simulink model "Planar_robot_3DoF_sim"  (R2023a)
settings: Solver=ode3  StartTime=0.0  StopTime=5  FixedStep=0.001  RelTol=1e-3
values from neighbouring files (symbols this model uses):
  amplitude = 20 + 20 * rand(1, num_links)'    [script.m]
  arm_length = [2 2 2]    [script.m]
  freq = 10 + 10 * rand(1, num_links)'    [script.m]
  radius = 0.00002    (= 2e-05)    [script.m]
  rho = 10000000    [script.m]
settings Model: Creator=wu_xw  LastModifiedBy=divij
settings SolverCC: AlgebraicLoopSolver=TrustRegion
settings DataIOCC: SaveFormat=Structure  SaveOutput=off  SignalLogging=off  DSMLogging=off  SaveTime=off  ReturnWorkspaceOutputs=off
settings OptimizationCC: DefaultParameterBehavior=Inlined  UseDivisionForNetSlopeComputation=on  GainParamInheritBuiltInType=on  UseFloatMulNetSlope=on  InlineInvariantSignals=on  ZeroExternalMemoryAtStartup=off  ZeroInternalMemoryAtStartup=off  EfficientFloat2IntCast=on  LifeSpan=1  OptimizeDataStoreBuffers=off  BusAssignmentInplaceUpdate=off
settings DebuggingCC: UnconnectedInputMsg=warning  UnconnectedOutputMsg=warning  UnconnectedLineMsg=warning  SFUnexpectedBacktrackingDiag=warning  SFNoUnconditionalDefaultTransitionDiag=warning  ArithmeticOperatorsInVariantConditions=warning
settings HardwareCC: ProdLongLongMode=on
settings ModelReferenceCC: EnableRefExpFcnMdlSchedulingChecks=on
settings SFSimCC: SimUseLocalCustomCode=off  MATLABDynamicMemAlloc=off  CustomCodeUndefinedFunction=UseInterfaceOnly
settings RTWCC: GenCodeOnly=on  PackageGeneratedCodeAndArtifacts=on  GenerateReport=on  RTWUseLocalCustomCode=off  Toolchain=Catkin  BuildConfiguration=Debug  LaunchReport=on  TargetLang=C++
settings CodeAppCC: ForceParamTrailComments=on  EnableCustomComments=on
settings GRTTargetCC: TargetLangStandard=C++11 (ISO)  CombineSignalStateStructs=on  MatFileLogging=off  CodeInterfacePackaging=C++ class  SupportVariableSizeSignals=on  MultiInstanceErrorCode=Warning

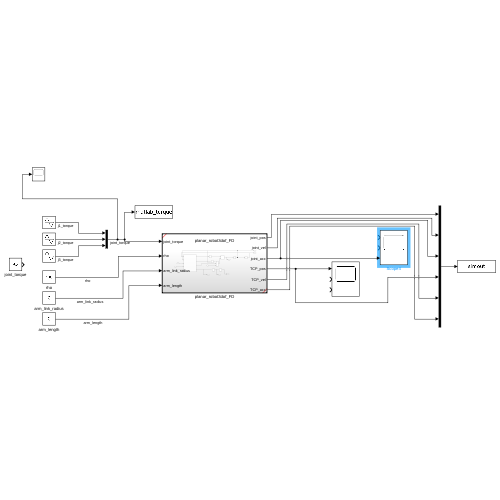
[thumbnail: Simulink's stored preview of the top-level diagram]
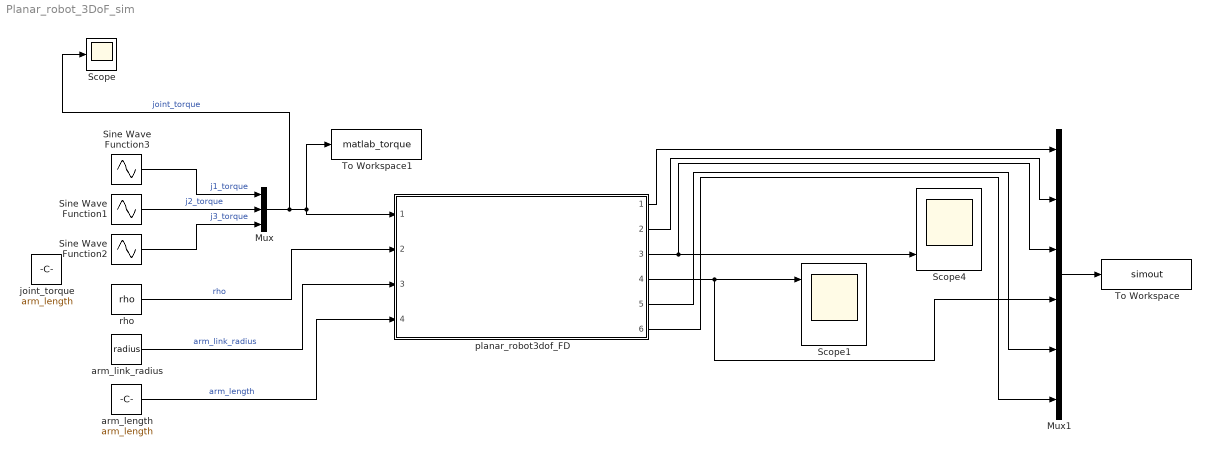
== system Planar_robot_3DoF_sim ==
  Mux : Mux  Inputs=3
  Mux1 : Mux  Inputs=6
  Scope : Scope
  Scope1 : Scope  NumInputPorts=3
  Scope4 : Scope  NumInputPorts=3
  Sine Wave Function1 : Sin  Amplitude=amplitude(2)  Frequency=freq(2)  SampleTime=0
  Sine Wave Function2 : Sin  Amplitude=amplitude(3)  Frequency=freq(3)  SampleTime=0
  Sine Wave Function3 : Sin  Amplitude=amplitude(1)  Frequency=freq(1)  SampleTime=0
  To Workspace : ToWorkspace  VariableName=simout  SaveFormat=Structure  SampleTime=-1
  To Workspace1 : ToWorkspace  VariableName=matlab_torque  SampleTime=-1
      settings: Save2DSignal=2-D array (concatenate along first dimension)
  arm_length : Constant  Value=arm_length  SampleTime=-1
  arm_link_radius : Constant  Value=radius  SampleTime=-1
  joint_torque : Constant  Value=arm_length  SampleTime=-1
  planar_robot3dof_FD : Subsystem  TreatAsAtomicUnit=on  ReferencedSubsystem=planar_robot3dof_FD
  rho : Constant  Value=rho  SampleTime=-1
  wires:
  Sine Wave Function1/1 -> Mux/2  "j2_torque"
  Sine Wave Function2/1 -> Mux/3  "j3_torque"
  arm_length/1 -> planar_robot3dof_FD/4  "arm_length"
  rho/1 -> planar_robot3dof_FD/2  "rho"
  arm_link_radius/1 -> planar_robot3dof_FD/3  "arm_link_radius"
  Mux/1 -> Scope/1, planar_robot3dof_FD/1, To Workspace1/1  "joint_torque"
  planar_robot3dof_FD/1 -> Mux1/1
  planar_robot3dof_FD/2 -> Mux1/2
  planar_robot3dof_FD/3 -> Scope4/3, Mux1/3
  planar_robot3dof_FD/4 -> Scope1/1, Mux1/4
  planar_robot3dof_FD/5 -> Mux1/5
  planar_robot3dof_FD/6 -> Mux1/6
  Mux1/1 -> To Workspace/1
  Sine Wave Function3/1 -> Mux/1  "j1_torque"
